simulink model "Correlation_Stream_Ex1"  (R2025a)
settings: Solver=ode4  StartTime=0.0  StopTime=5  RelTol=1e-3
PreLoadFcn:
  | init
undefined symbols (not defined in the file): DUT, i, L, stream_correlation_smoke, Valid, viva1596, xcvc1902
libraries: dspsrcs4 x2, aieDSP x1, vmcUtilities x1
settings Model: Creator=sais  LastModifiedBy=sdegala

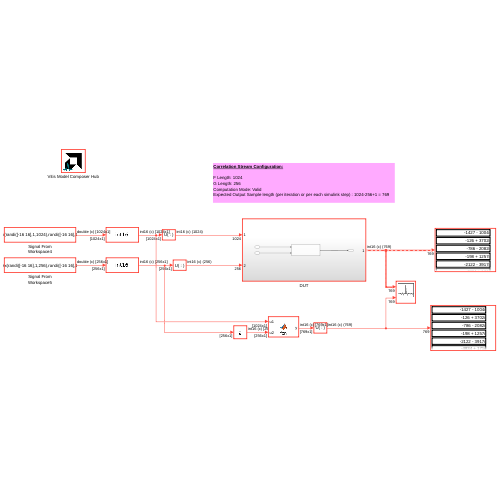
[thumbnail: Simulink's stored preview of the top-level diagram]
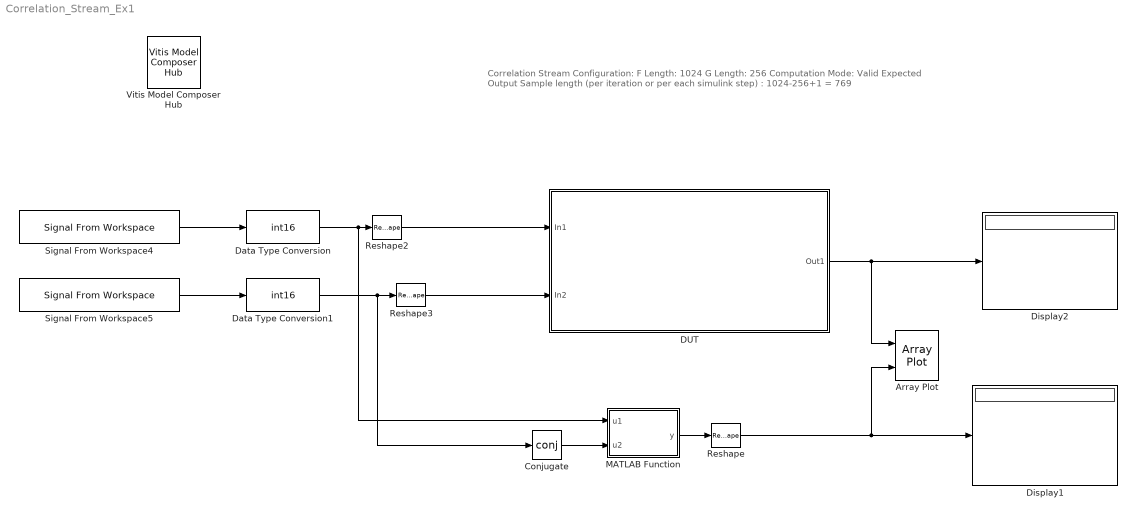
== system Correlation_Stream_Ex1 ==
  note: Correlation Stream Configuration:
      |
      | F Length: 1024
      | G Length: 256
      | Computation Mode: Valid
      | Expected Output Sample length (per iteration or per each simulink step) : 1024-256+1 = 769
  Array Plot : ArrayPlot  NumInputPorts=2  WindowPosition=[169.000000,231.000000,800.000000,500.000000,]  Visible=on  ScopeFrameLocation=window  YLimits=[-9400.75 10596.75]  ShowLegend=on
  Conjugate : Math  Operator=conj  SignedPower=on  RndMeth=Zero
  DUT : Subsystem
  Data Type Conversion : DataTypeConversion  OutDataTypeStr=int16  SaturateOnIntegerOverflow=off  RndMeth=Floor
  Data Type Conversion1 : DataTypeConversion  OutDataTypeStr=int16  SaturateOnIntegerOverflow=off  RndMeth=Floor
  Display1 : Display
  Display2 : Display
  MATLAB Function : MATLAB Function  TreatAsAtomicUnit=on
  Reshape : Reshape
  Reshape2 : Reshape
  Reshape3 : Reshape
  Signal From Workspace4 : dspsrcs4/Signal From Workspace  X=complex(randi([-16 16],1,1024),randi([-16 16],1,1024))  Ts=1  nsamps=1024  OutputAfterFinalValue=Setting to zero  ignoreOrWarnInputAndFrameLengths=off  OutputFrames=off
  Signal From Workspace5 : dspsrcs4/Signal From Workspace  X=complex(randi([-16 16],1,256),randi([-16 16],1,256))  Ts=1*(1024/256)  nsamps=256  OutputAfterFinalValue=Setting to zero  ignoreOrWarnInputAndFrameLengths=off  OutputFrames=off
  Vitis Model Composer Hub : vmcUtilities/Vitis Model Composer Hub  Tag=genX  CodeGeneration=off  SubsystemName=DUT  BlockHierPath=stream_correlation_smoke/DUT  CompilationType=HDLCompilation  SubsystemType=AIENode  ExportTypeV2=IP Catalog  AIEArrayConfig=Use entire AIE array  StartColumn=1  NumberOfColumns=1  TargetDirectory=./code_2iterations  exportDesign=off  analyzeDesign=on  validateDesignOnHw=off  ExportType=AI Engines  IpVendor=xilinx.com  IpLibrary=hls  IpVersion=1.0  IpHWLanguage=Verilog  AieCompilerOptions={}  AieSimulatorOptions={}  CreateTestbench=on  TestbenchStackSize=10  RunRtlSim=off  RunCSim=off  RunAieSim=off  enableSimulationTimeout=on  enableGraphIterations=on  AieSimTimeout=50000  AieGraphIterations=-1  RunAieSimProfiling=off  LaunchVitisAnalyzer=off  PlotOutput=off  RunX86Sim=off  X86SimTimeout=10  GenHwImage=off  GenLibadfXo=off  GenHwValidationCode=off  PlatformType=Not Specified  HwSystemType=Baremetal  HwValidationTarget=hw  ProjDevice=xcvc1902-viva1596-1LHP-i-L  ProjDevicePart=xcvc1902-viva1596-1LHP-i-L  AIEType=AIE  SamplePeriod=-1  ClockFrequency=200  DataPathParallelism=1  xilinxfamily=versalaicore  part=xcvc1902  speed=-1LHP-i-L  package=viva1596  directory=./netlist  testbench=off  incr_netlist=off  synthesis_tool=Vivado  clock_wrapper=Clock Enables  dbl_ovrd=According to Block Masks  dcm_input_clock_period=10  sysclk_period=10  simulink_period=1  eval_field=0  IPInfoJsonString="{\"DUTSubsystemName\":\"DUT\",\"AIESubsystem\":{\"SubsystemName\":\"DUT\",\"TargetDirectory\":\"./code_2iterations\",\"AIEArrayConfig\":\"Use entire AIE array\",\"StartColumn\":\"0\",\"NumberOfColumns\":\"1\"},\"SubsystemTag\":\"AIENode\"}"  LogFileName=/proj/xhdhdstaff5/sdegala/Head1/HEAD/2026_1_Work/code_2iterations/model_composer.log  NThreads=4  IPConfigFile=/tmp/vmctmp-11698742404697829623/stream_correlation_smoke_ipconfig.json
  wires:
  Conjugate/1 -> MATLAB Function/2(u2)
  MATLAB Function/1(y) -> Reshape/1
  Reshape2/1 -> DUT/1(In1)
  Reshape3/1 -> DUT/2(In2)
  DUT/1(Out1) -> Display2/1, Array Plot/1
  Reshape/1 -> Display1/1, Array Plot/2
  Signal From Workspace4/1 -> Data Type Conversion/1
  Signal From Workspace5/1 -> Data Type Conversion1/1
  Data Type Conversion/1 -> MATLAB Function/1(u1), Reshape2/1
  Data Type Conversion1/1 -> Conjugate/1, Reshape3/1

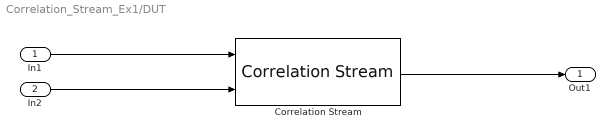
== system Correlation_Stream_Ex1/DUT ==
  In1 : Inport
  In2 : Inport  Port=2
  Correlation Stream : aieDSP/Correlation Stream  AIE_VARIANT=1  api=1  data_type_f=cint16  data_type_g=cint16  data_type_out=cint16  function_type=0  compute_mode=Valid (2)  f_sample_size=1024  g_sample_size=256  USE_RTP_VECTOR_LENGTHS=off  num_frames=1  shift_output=0  rnd_mode=Floor  sat_mode=None  no_of_kernels=1  casc_length=8  blockJsonConstraints=[]  blockJsonConstraintsInternal=[]  spec=vmc_stream_corr.json  SerializedMaskParamNames=[]  SerializedMaskParamValues=[]  SerializedMaskParamVisibilities=[]  block_type=Correlation Stream  SerializedMaskParamDataypes=uint|uint|typename|typename|typename|uint|uint|uint|uint|uint|uint|uint|uint|uint|uint|uint  SerializedMaskParamEnumStrArr=0|0|0|0|0|0|Valid (2)|0|0|0|0|0|Floor,Ceiling,Round to positive infinity,Round to negative infinity,Round symmetrical to infinity,Round symmetrical to zero,Round convergent to even,Round convergent to odd|None,Saturate,Symmetric|0|0  SerializedMaskParamEnumValArr=0|0|0|0|0|0|2|0|0|0|0|0|0,1,2,3,4,5,6,7|0,1,3|0|0  SerializedMaskParamVectorArr=0|0|0|0|0|0|0|0|0|0|0|0|0|0|0|0  SerializedMaskParamKeys=AIE_VARIANT|TP_API|TT_DATA_F|TT_DATA_G|TT_DATA_OUT|TP_FUNCT_TYPE|TP_COMPUTE_MODE|TP_F_LEN|TP_G_LEN|TP_USE_RTP_VECTOR_LENGTHS|TP_NUM_FRAMES|TP_SHIFT|TP_RND|TP_SAT|TP_PHASES|TP_CASC_LEN
  Out1 : Outport
  wires:
  In1/1 -> Correlation Stream/1
  Correlation Stream/1 -> Out1/1
  In2/1 -> Correlation Stream/2

== matlab function Correlation_Stream_Ex1/MATLAB Function ==
  data: u1 input; y output; u2 input
function y = fcn(u1,u2)

y = int16(conv(u1,flip(u2),"valid"));
